simulink model "psocarea"  (R2024b)
settings: Solver=VariableStepAuto  StartTime=0.0  StopTime=10.0  RelTol=1e-3
settings Model: Creator=ASUS  LastModifiedBy=ASUS

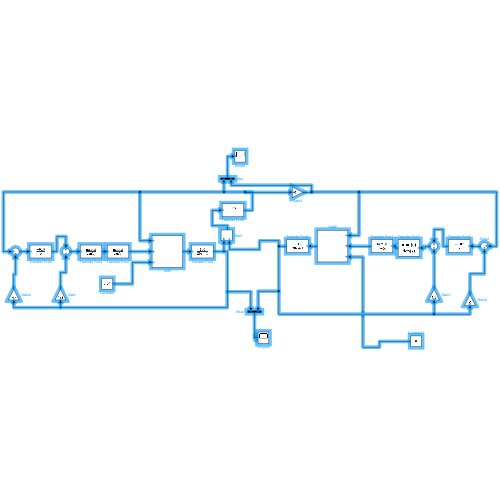
[thumbnail: Simulink's stored preview of the top-level diagram]
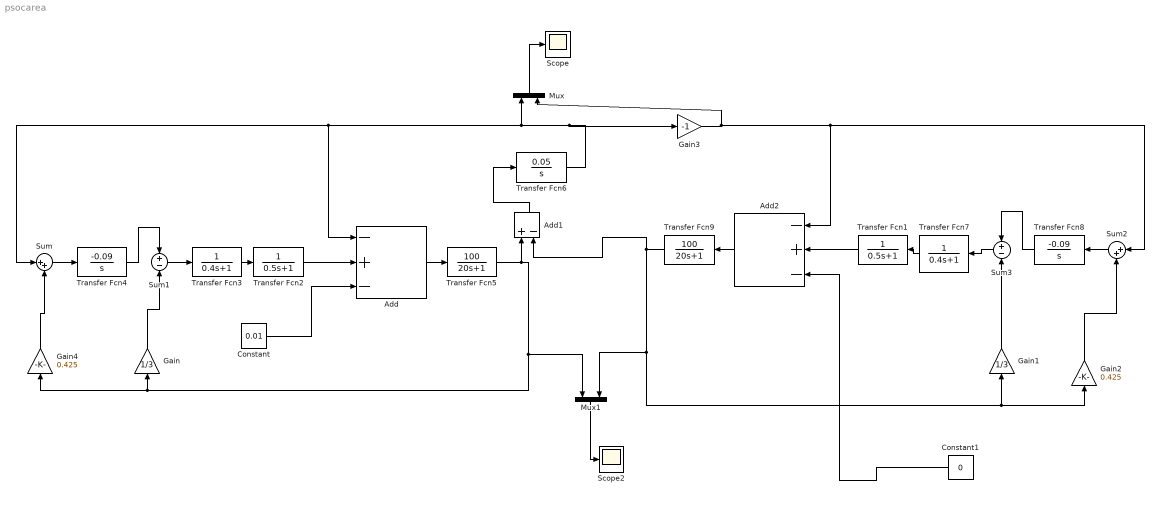
== system psocarea ==
  Add : Sum  Inputs=-+-
  Add1 : Sum  Inputs=+-
  Add2 : Sum  Inputs=-+-
  Constant : Constant  Value=0.01
  Constant1 : Constant  Value=0
  Gain : Gain  Gain=1/3
  Gain1 : Gain  Gain=1/3
  Gain2 : Gain  Gain=0.425
  Gain3 : Gain  Gain=-1
  Gain4 : Gain  Gain=0.425
  Mux : Mux  Inputs=2
  Mux1 : Mux  Inputs=2
  Scope : Scope
  Scope2 : Scope
  Sum : Sum  Inputs=|++
  Sum1 : Sum  Inputs=+-
  Sum2 : Sum  Inputs=|++
  Sum3 : Sum  Inputs=+-
  Transfer Fcn1 : TransferFcn  Denominator=[0.5 1]
  Transfer Fcn2 : TransferFcn  Denominator=[0.5 1]
  Transfer Fcn3 : TransferFcn  Denominator=[0.4 1]
  Transfer Fcn4 : TransferFcn  Numerator=[-0.09]  Denominator=[1 0]
  Transfer Fcn5 : TransferFcn  Numerator=[100]  Denominator=[20 1]
  Transfer Fcn6 : TransferFcn  Numerator=[0.05]  Denominator=[1 0]  ParameterTunability=Optimized
  Transfer Fcn7 : TransferFcn  Denominator=[0.4 1]
  Transfer Fcn8 : TransferFcn  Numerator=[-0.09]  Denominator=[1 0]
  Transfer Fcn9 : TransferFcn  Numerator=[100]  Denominator=[20 1]
  wires:
  Mux/1 -> Scope/1
  Transfer Fcn6/1 -> Gain3/1, Add/1, Sum/1, Mux/1
  Sum/1 -> Transfer Fcn4/1
  Transfer Fcn4/1 -> Sum1/1
  Sum1/1 -> Transfer Fcn3/1
  Transfer Fcn3/1 -> Transfer Fcn2/1
  Transfer Fcn2/1 -> Add/2
  Constant/1 -> Add/3
  Add1/1 -> Transfer Fcn6/1
  Add/1 -> Transfer Fcn5/1
  Gain4/1 -> Sum/2
  Transfer Fcn5/1 -> Add1/1, Mux1/1, Gain/1, Gain4/1
  Gain/1 -> Sum1/2
  Mux1/1 -> Scope2/1
  Gain1/1 -> Sum3/2
  Transfer Fcn9/1 -> Add1/2, Mux1/2, Gain1/1, Gain2/1
  Sum3/1 -> Transfer Fcn7/1
  Constant1/1 -> Add2/3
  Transfer Fcn8/1 -> Sum3/1
  Transfer Fcn7/1 -> Transfer Fcn1/1
  Transfer Fcn1/1 -> Add2/2
  Gain2/1 -> Sum2/2
  Sum2/1 -> Transfer Fcn8/1
  Add2/1 -> Transfer Fcn9/1
  Gain3/1 -> Add2/1, Sum2/1, Mux/2
